simulink model "HHM_2"  (R2018a)
settings: Solver=VariableStepAuto  StartTime=0.0  StopTime=40.0  RelTol=1e-3
values from neighbouring files (symbols this model uses):
  Cm = 1*10^-6    (= 1e-06)    [HHM_3.m]
  Ek = -72*10^-3    (= -0.072)    [HHM_3.m]
  El = -49.4*10^-3    (= -0.0494)    [HHM_3.m]
  Ena = 55*10^-3    (= 0.055)    [HHM_3.m]
  GKbar = 36*10^-3    (= 0.036)    [HHM_3.m]
  GL = 0.3*10^-3    (= 0.0003)    [HHM_3.m]
  GNabar = 120*10^-3    (= 0.12)    [HHM_3.m]
  K = 30*10^-6    (= 3e-05)    [HHM_3.m]
  K2 = 0*50*10^-6    (= 0)    [HHM_3.m]
  sti = 16    [HHM_3.m]
  sti2 = 25    [HHM_3.m]
  t0 = 10*10^-3    (= 0.01)    [HHM_3.m]
  t02 = 15*10^-3    (= 0.015)    [HHM_3.m]
settings Model: Creator=hp  LastModifiedBy=hp

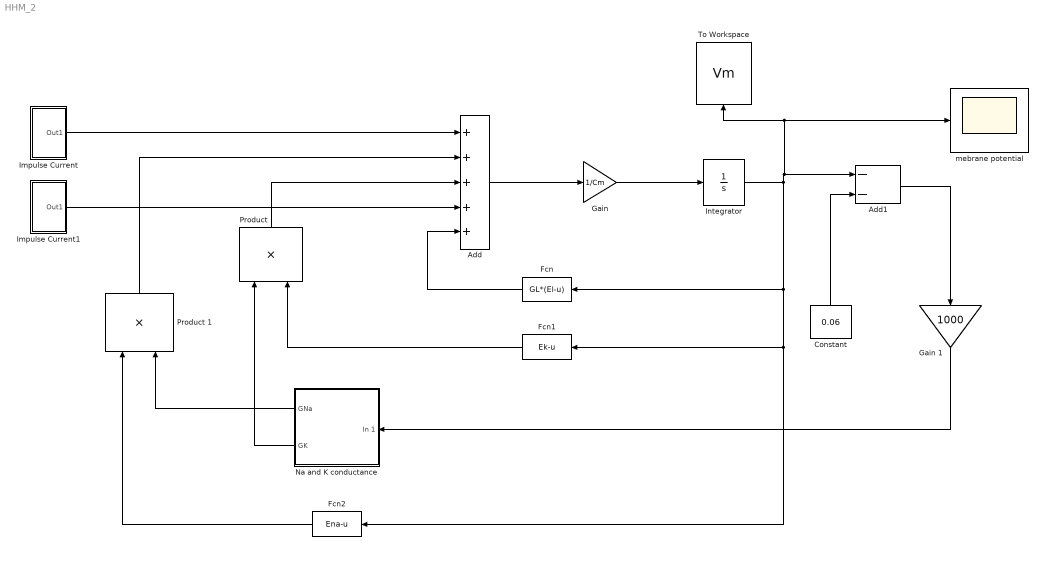
== system HHM_2 ==
  "Add " : Sum  Inputs=+++++
  "Add1 " : Sum  Inputs=--
  "Constant " : Constant  Value=0.06
  "Fcn " : Fcn  Expr=GL*(El-u)
  "Fcn1 " : Fcn  Expr=Ek-u
  "Fcn2 " : Fcn  Expr=Ena-u
  "Gain " : Gain  Gain=1/Cm
  Gain 1 : Gain  Gain=1000
  Impulse Current : Subsystem
  Impulse Current1 : Subsystem
  Integrator : Integrator  InitialCondition=-.06
  Na and K conductance : Subsystem
  "Product " : Product
  Product 1 : Product
  "To Workspace " : ToWorkspace  VariableName=Vm  SaveFormat=Timeseries  SampleTime=-1
  mebrane potential : Scope
  wires:
  Impulse Current/1(Out1) -> "Add "/1
  Gain 1/1 -> Na and K conductance/1(In 1)
  Na and K conductance/1("GNa ") -> Product 1/2
  Na and K conductance/2("GK ") -> "Product "/1
  "Fcn2 "/1 -> Product 1/1
  Impulse Current1/1(Out1) -> "Add "/4
  Product 1/1 -> "Add "/2
  "Product "/1 -> "Add "/3
  "Add "/1 -> "Gain "/1
  "Gain "/1 -> Integrator/1
  "Constant "/1 -> "Add1 "/2
  "Add1 "/1 -> Gain 1/1
  Integrator/1 -> "Add1 "/1, mebrane potential/1, "To Workspace "/1, "Fcn2 "/1, "Fcn1 "/1, "Fcn "/1
  "Fcn "/1 -> "Add "/5
  "Fcn1 "/1 -> "Product "/2

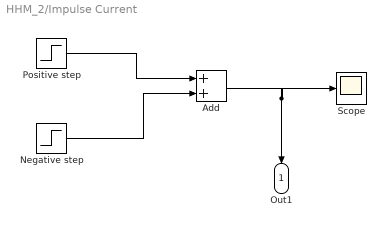
== system HHM_2/Impulse Current ==
  Add : Sum
  Negative step : Step  Time=sti+t0  After=-K  SampleTime=0
  Positive step : Step  Time=sti  After=K  SampleTime=0
  Scope : Scope
  Out1 : Outport
  wires:
  Add/1 -> Scope/1, Out1/1
  Positive step/1 -> Add/1
  Negative step/1 -> Add/2

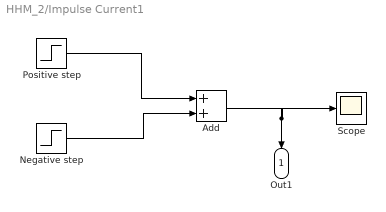
== system HHM_2/Impulse Current1 ==
  Add : Sum
  Negative step : Step  Time=sti2+t02  After=-K2  SampleTime=0
  Positive step : Step  Time=sti2  After=K2  SampleTime=1
  Scope : Scope
  Out1 : Outport
  wires:
  Add/1 -> Scope/1, Out1/1
  Negative step/1 -> Add/2
  Positive step/1 -> Add/1

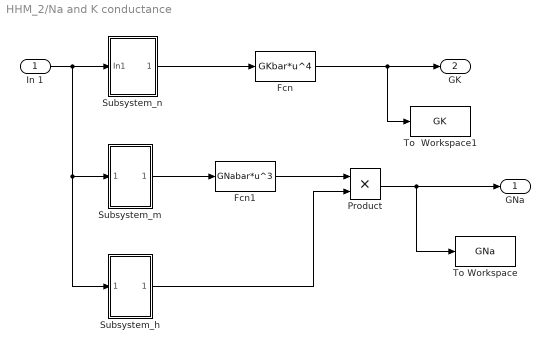
== system HHM_2/Na and K conductance ==
  In 1 : Inport
  "Fcn " : Fcn  Expr=GKbar*u^4
  "Fcn1 " : Fcn  Expr=GNabar*u^3
  "Product " : Product
  Subsystem_h : Subsystem
  Subsystem_m : Subsystem
  Subsystem_n : Subsystem
  To  Workspace1 : ToWorkspace  VariableName=GK  SaveFormat=Timeseries  SampleTime=-1
  "To Workspace " : ToWorkspace  VariableName=GNa  SaveFormat=Timeseries  SampleTime=-1
  "GNa " : Outport
  "GK " : Outport  Port=2
  wires:
  In 1/1 -> Subsystem_n/1(In1), Subsystem_h/1(In1), Subsystem_m/1(In1)
  Subsystem_m/1(Out2) -> "Fcn1 "/1
  "Product "/1 -> "GNa "/1, "To Workspace "/1
  "Fcn "/1 -> "GK "/1, To  Workspace1/1
  "Fcn1 "/1 -> "Product "/1
  Subsystem_h/1(Out2) -> "Product "/2
  Subsystem_n/1(Out2) -> "Fcn "/1

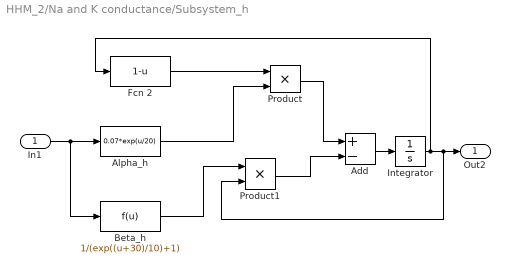
== system HHM_2/Na and K conductance/Subsystem_h ==
  In1 : Inport
  " Integrator" : Integrator
  "Add " : Sum  Inputs=+-
  Alpha_h : Fcn  Expr=0.07*exp(u/20)
  Beta_h : Fcn  Expr=1/(exp((u+30)/10)+1)
  Fcn 2 : Fcn  Expr=1-u
  "Product " : Product
  "Product1 " : Product
  Out2 : Outport
  wires:
  Beta_h/1 -> "Product1 "/1
  Fcn 2/1 -> "Product "/1
  In1/1 -> Beta_h/1, Alpha_h/1
  " Integrator"/1 -> Out2/1, "Product1 "/2, Fcn 2/1
  "Add "/1 -> " Integrator"/1
  Alpha_h/1 -> "Product "/2
  "Product "/1 -> "Add "/1
  "Product1 "/1 -> "Add "/2

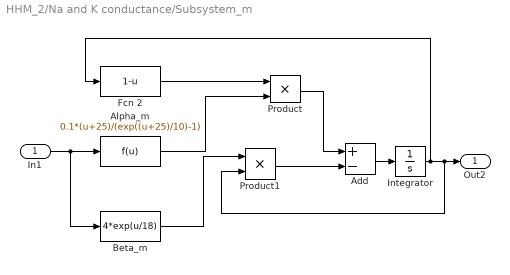
== system HHM_2/Na and K conductance/Subsystem_m ==
  In1 : Inport
  "Add " : Sum  Inputs=+-
  Alpha_m : Fcn  Expr=0.1*(u+25)/(exp((u+25)/10)-1)
  Beta_m : Fcn  Expr=4*exp(u/18)
  Fcn 2 : Fcn  Expr=1-u
  "Integrator " : Integrator
  "Product " : Product
  "Product1 " : Product
  Out2 : Outport
  wires:
  Beta_m/1 -> "Product1 "/1
  Fcn 2/1 -> "Product "/1
  In1/1 -> Beta_m/1, Alpha_m/1
  "Integrator "/1 -> Out2/1, "Product1 "/2, Fcn 2/1
  "Add "/1 -> "Integrator "/1
  Alpha_m/1 -> "Product "/2
  "Product "/1 -> "Add "/1
  "Product1 "/1 -> "Add "/2

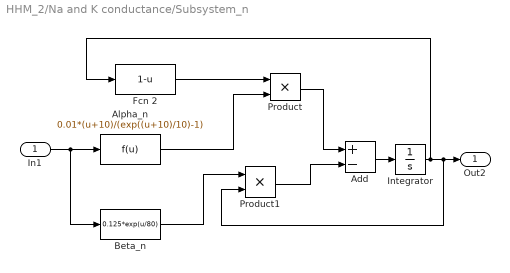
== system HHM_2/Na and K conductance/Subsystem_n ==
  In1 : Inport
  "Add " : Sum  Inputs=+-
  Alpha_n : Fcn  Expr=0.01*(u+10)/(exp((u+10)/10)-1)
  Beta_n : Fcn  Expr=0.125*exp(u/80)
  Fcn 2 : Fcn  Expr=1-u
  "Integrator " : Integrator
  "Product " : Product
  "Product1 " : Product
  Out2 : Outport
  wires:
  Beta_n/1 -> "Product1 "/1
  Fcn 2/1 -> "Product "/1
  In1/1 -> Beta_n/1, Alpha_n/1
  "Integrator "/1 -> Out2/1, "Product1 "/2, Fcn 2/1
  "Add "/1 -> "Integrator "/1
  Alpha_n/1 -> "Product "/2
  "Product "/1 -> "Add "/1
  "Product1 "/1 -> "Add "/2
